simulink model "ft_sensor_debug_iCubGenova03"  (Simulink 8.3)
settings: Solver=FixedStepDiscrete  StartTime=0.0  StopTime=inf  RelTol=1e-3
libraries: WBCLibrary x8
settings Model: Creator=pegua  LastModifiedBy=pegua
settings DataIOCC: SignalLoggingSaveFormat=Dataset
settings DebuggingCC: UnderspecifiedInitializationDetection=Simplified  StateNameClashWarn=none
settings GRTTargetCC: CombineOutputUpdateFcns=on  GRTInterface=off

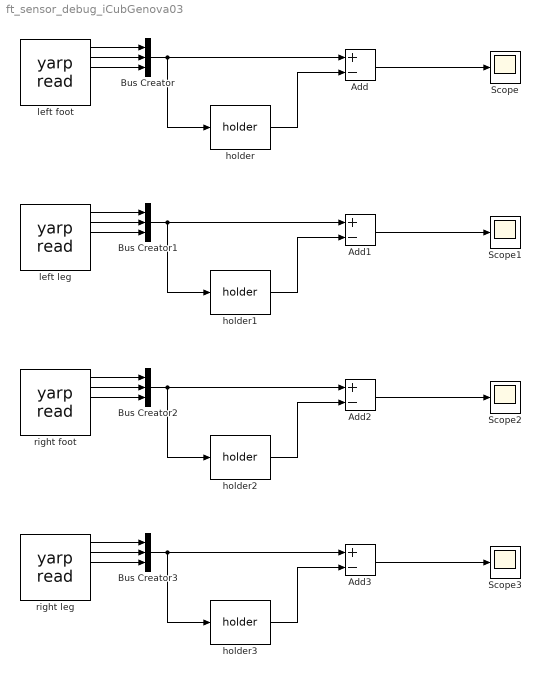
== system ft_sensor_debug_iCubGenova03 ==
  Add{,1..3} (4 alike) : Sum  Inputs=+-
  Bus Creator{,1..3} (4 alike) : BusCreator  Inputs=3
  Scope{,1..3} (4 alike) : Scope
      Scope settings: YMin=-4.5  YMax=0
      Scope1 settings: YMin=-45  YMax=0
      Scope2 settings: YMin=-4  YMax=0.5  SaveName=ScopeData2
      Scope3 settings: YMin=-45  YMax=0  SaveName=ScopeData3
  holder{,1..3} (4 alike) : WBCLibrary/Utilities/holder
  "left foot " : WBCLibrary/Utilities/yarp read  from=['/icub/left_foot/analog:o']  to='...'  num=6
  "left leg " : WBCLibrary/Utilities/yarp read  from=['/icub/left_leg/analog:o']  to='...'  num=6
  right foot : WBCLibrary/Utilities/yarp read  from=['/icub/right_foot/analog:o']  to='...'  num=6
  right leg : WBCLibrary/Utilities/yarp read  from=['/icub/right_leg/analog:o']  to='...'  num=6
  wires:
  "left foot "/1 -> Bus Creator/1
  "left foot "/2 -> Bus Creator/2
  "left foot "/3 -> Bus Creator/3
  Bus Creator/1 -> Add/1, holder/1
  holder/1 -> Add/2
  Add/1 -> Scope/1
  "left leg "/1 -> Bus Creator1/1
  "left leg "/2 -> Bus Creator1/2
  "left leg "/3 -> Bus Creator1/3
  Bus Creator1/1 -> Add1/1, holder1/1
  holder1/1 -> Add1/2
  Add1/1 -> Scope1/1
  right foot/1 -> Bus Creator2/1
  right foot/2 -> Bus Creator2/2
  right foot/3 -> Bus Creator2/3
  Bus Creator2/1 -> Add2/1, holder2/1
  holder2/1 -> Add2/2
  Add2/1 -> Scope2/1
  right leg/1 -> Bus Creator3/1
  right leg/2 -> Bus Creator3/2
  right leg/3 -> Bus Creator3/3
  Bus Creator3/1 -> Add3/1, holder3/1
  holder3/1 -> Add3/2
  Add3/1 -> Scope3/1
